simulink model "Trajektorienfolgeregelung_test"  (R2020a)
settings: Solver=ode1  StartTime=0.0  StopTime=3.5  FixedStep=0.01  RelTol=1e-10
undefined symbols (not defined in the file or in its folder): simparams
libraries: dspfdesign x3
settings Model: Creator=Frederik  LastModifiedBy=Frederik

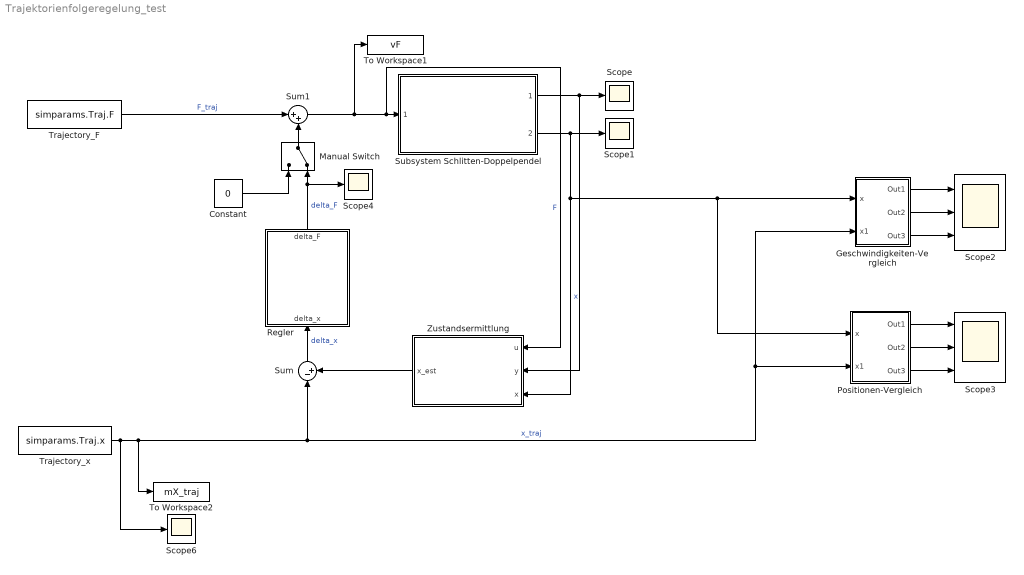
== system Trajektorienfolgeregelung_test ==
  Constant : Constant  Value=0
  Geschwindigkeiten-Vergleich : Subsystem
  Manual Switch : ManualSwitch  CurrentSetting=0
  Positionen-Vergleich : Subsystem
  Regler : Subsystem  mask{RegData=simparams.TrajRegDataF}
      mask prompts: RegData "TrajRegDataF"
  Scope{,1,4,6} (4 alike) : Scope
  Scope2 : Scope  NumInputPorts=3
  Scope3 : Scope  NumInputPorts=3
  Subsystem Schlitten-Doppelpendel : Subsystem  ReferencedSubsystem=SchlittenPendel  params=simparams.gesamtmodell.schlittenpendel
  Sum : Sum  Inputs=|-+
  Sum1 : Sum  Inputs=|++
  To Workspace1 : ToWorkspace  VariableName=vF  SaveFormat=Timeseries  SampleTime=-1
  To Workspace2 : ToWorkspace  VariableName=mX_traj  SaveFormat=Timeseries  SampleTime=-1
  Trajectory_F : FromWorkspace  VariableName=simparams.Traj.F  Interpolate=off  OutputAfterFinalValue=Setting to zero
  Trajectory_x : FromWorkspace  VariableName=simparams.Traj.x  Interpolate=off  OutputAfterFinalValue=Setting to zero
  Zustandsermittlung : Subsystem  Variant=on  VariantControl=Choice  PropagateVariantConditions=on  mask{BeoData=simparams.TrajRegDataF, xtype=Zustandsmessung}
      mask prompts: BeoData "Beobachter"; xtype "Zustandsermittlung"
      mask TypeOptions xtype: Zustandsmessung | Beobachter | Differenzieren
  wires:
  Subsystem Schlitten-Doppelpendel/1 -> Zustandsermittlung/2(y), Scope/1
  Trajectory_x/1 -> Sum/1, Positionen-Vergleich/2(x1), Geschwindigkeiten-Vergleich/2(x1), To Workspace2/1, Scope6/1  "x_traj"
  Trajectory_F/1 -> Sum1/1  "F_traj"
  Sum1/1 -> To Workspace1/1, Zustandsermittlung/1(u), Subsystem Schlitten-Doppelpendel/1  "F"
  Manual Switch/1 -> Sum1/2
  Constant/1 -> Manual Switch/1
  Sum/1 -> Regler/1(delta_x)  "delta_x"
  Regler/1(delta_F) -> Scope4/1, Manual Switch/2  "delta_F"
  Geschwindigkeiten-Vergleich/1(Out1) -> Scope2/1
  Geschwindigkeiten-Vergleich/2(Out2) -> Scope2/2
  Geschwindigkeiten-Vergleich/3(Out3) -> Scope2/3
  Positionen-Vergleich/1(Out1) -> Scope3/1
  Positionen-Vergleich/2(Out2) -> Scope3/2
  Positionen-Vergleich/3(Out3) -> Scope3/3
  Subsystem Schlitten-Doppelpendel/2 -> Zustandsermittlung/3(x), Positionen-Vergleich/1(x), Geschwindigkeiten-Vergleich/1(x), Scope1/1  "x"
  Zustandsermittlung/1(x_est) -> Sum/2

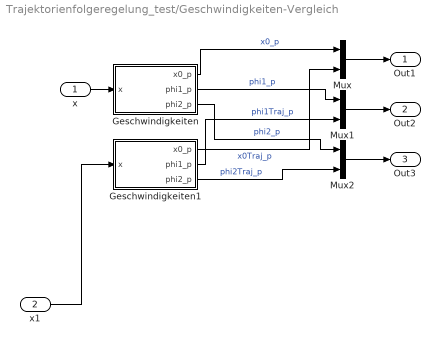
== system Trajektorienfolgeregelung_test/Geschwindigkeiten-Vergleich ==
  x : Inport
  x1 : Inport  Port=2
  Geschwindigkeiten : Subsystem
  Geschwindigkeiten1 : Subsystem
  Mux : Mux  Inputs=2
  Mux1 : Mux  Inputs=2
  Mux2 : Mux  Inputs=2
  Out1 : Outport
  Out2 : Outport  Port=2
  Out3 : Outport  Port=3
  wires:
  Geschwindigkeiten/1(x0_p) -> Mux/1  "x0_p"
  x/1 -> Geschwindigkeiten/1(x)
  Mux1/1 -> Out2/1
  Geschwindigkeiten1/2(phi1_p) -> Mux1/2  "phi1Traj_p"
  Geschwindigkeiten/3(phi2_p) -> Mux2/1  "phi2_p"
  Geschwindigkeiten1/3(phi2_p) -> Mux2/2  "phi2Traj_p"
  x1/1 -> Geschwindigkeiten1/1(x)
  Mux2/1 -> Out3/1
  Geschwindigkeiten1/1(x0_p) -> Mux/2  "x0Traj_p"
  Geschwindigkeiten/2(phi1_p) -> Mux1/1  "phi1_p"
  Mux/1 -> Out1/1

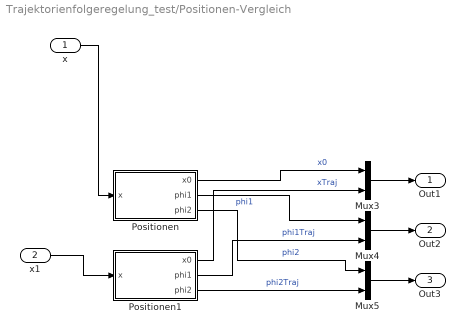
== system Trajektorienfolgeregelung_test/Positionen-Vergleich ==
  x : Inport
  x1 : Inport  Port=2
  Mux3 : Mux  Inputs=2
  Mux4 : Mux  Inputs=2
  Mux5 : Mux  Inputs=2
  Positionen : Subsystem
  Positionen1 : Subsystem
  Out1 : Outport
  Out2 : Outport  Port=2
  Out3 : Outport  Port=3
  wires:
  Positionen/3(phi2) -> Mux5/1  "phi2"
  Mux3/1 -> Out1/1
  Positionen1/3(phi2) -> Mux5/2  "phi2Traj"
  x1/1 -> Positionen1/1(x)
  Mux5/1 -> Out3/1
  Mux4/1 -> Out2/1
  Positionen1/1(x0) -> Mux3/2  "xTraj"
  Positionen1/2(phi1) -> Mux4/2  "phi1Traj"
  Positionen/1(x0) -> Mux3/1  "x0"
  Positionen/2(phi1) -> Mux4/1  "phi1"
  x/1 -> Positionen/1(x)

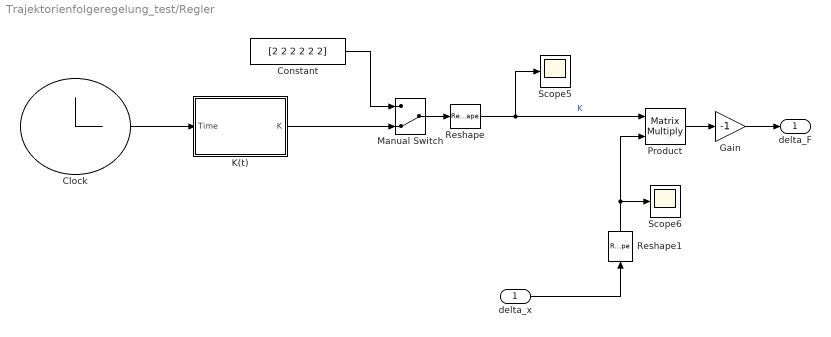
== system Trajektorienfolgeregelung_test/Regler ==
  delta_x : Inport
  Clock : Clock
  Constant : Constant  Value=[2 2 2 2 2 2]
  Gain : Gain  Gain=-1
  K(t) : Subsystem
  Manual Switch : ManualSwitch  CurrentSetting=0
  Product : Product  Multiplication=Matrix(*)
  Reshape : Reshape  OutputDimensionality=Row vector (2-D)
  Reshape1 : Reshape  OutputDimensionality=Column vector (2-D)
  Scope5 : Scope
  Scope6 : Scope
  delta_F : Outport
  wires:
  Product/1 -> Gain/1
  Reshape1/1 -> Product/2, Scope6/1
  Reshape/1 -> Scope5/1, Product/1  "K"
  delta_x/1 -> Reshape1/1
  Constant/1 -> Manual Switch/1
  Gain/1 -> delta_F/1
  Manual Switch/1 -> Reshape/1
  Clock/1 -> K(t)/1(Time)
  K(t)/1(K) -> Manual Switch/2

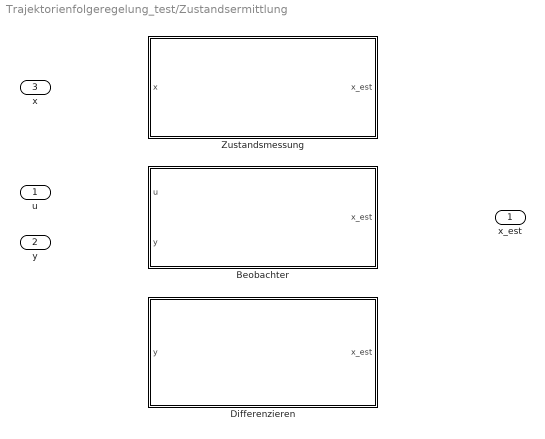
== system Trajektorienfolgeregelung_test/Zustandsermittlung ==
  u : Inport
  y : Inport  Port=2
  x : Inport  Port=3
  Beobachter : Subsystem  VariantControl=simparams.Zustandsermittlung==2
  Differenzieren : Subsystem  VariantControl=simparams.Zustandsermittlung==3
  Zustandsmessung : Subsystem  VariantControl=simparams.Zustandsermittlung==1
  x_est : Outport

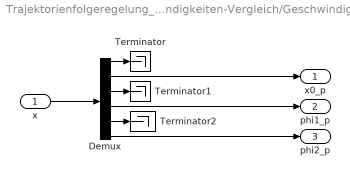
== system Trajektorienfolgeregelung_test/Geschwindigkeiten-Vergleich/Geschwindigkeiten ==
  x : Inport
  Demux : Demux  Outputs=6
  Terminator : Terminator
  Terminator1 : Terminator
  Terminator2 : Terminator
  x0_p : Outport
  phi1_p : Outport  Port=2
  phi2_p : Outport  Port=3
  wires:
  Demux/4 -> phi1_p/1
  Demux/2 -> x0_p/1
  Demux/5 -> Terminator2/1
  x/1 -> Demux/1
  Demux/3 -> Terminator1/1
  Demux/1 -> Terminator/1
  Demux/6 -> phi2_p/1

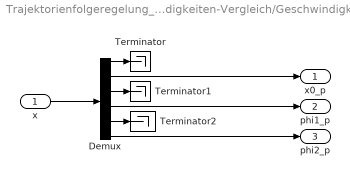
== system Trajektorienfolgeregelung_test/Geschwindigkeiten-Vergleich/Geschwindigkeiten1 ==
  x : Inport
  Demux : Demux  Outputs=6
  Terminator : Terminator
  Terminator1 : Terminator
  Terminator2 : Terminator
  x0_p : Outport
  phi1_p : Outport  Port=2
  phi2_p : Outport  Port=3
  wires:
  Demux/4 -> phi1_p/1
  Demux/2 -> x0_p/1
  Demux/5 -> Terminator2/1
  x/1 -> Demux/1
  Demux/3 -> Terminator1/1
  Demux/1 -> Terminator/1
  Demux/6 -> phi2_p/1

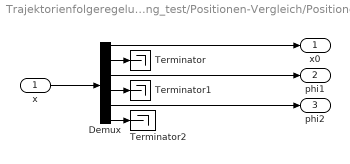
== system Trajektorienfolgeregelung_test/Positionen-Vergleich/Positionen ==
  x : Inport
  Demux : Demux  Outputs=6
  Terminator : Terminator
  Terminator1 : Terminator
  Terminator2 : Terminator
  x0 : Outport
  phi1 : Outport  Port=2
  phi2 : Outport  Port=3
  wires:
  Demux/3 -> phi1/1
  Demux/1 -> x0/1
  x/1 -> Demux/1
  Demux/5 -> phi2/1
  Demux/2 -> Terminator/1
  Demux/4 -> Terminator1/1
  Demux/6 -> Terminator2/1

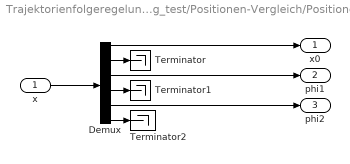
== system Trajektorienfolgeregelung_test/Positionen-Vergleich/Positionen1 ==
  x : Inport
  Demux : Demux  Outputs=6
  Terminator : Terminator
  Terminator1 : Terminator
  Terminator2 : Terminator
  x0 : Outport
  phi1 : Outport  Port=2
  phi2 : Outport  Port=3
  wires:
  Demux/3 -> phi1/1
  Demux/1 -> x0/1
  x/1 -> Demux/1
  Demux/5 -> phi2/1
  Demux/2 -> Terminator/1
  Demux/4 -> Terminator1/1
  Demux/6 -> Terminator2/1

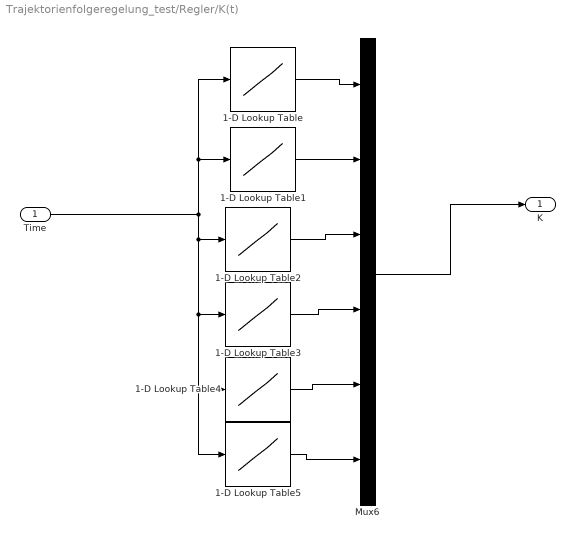
== system Trajektorienfolgeregelung_test/Regler/K(t) ==
  Time : Inport
  1-D Lookup Table : Lookup_n-D  NumberOfTableDimensions=1  BreakpointsForDimension1=RegData.T.data  Table=RegData.K.data(:,1)  InternalRulePriority=Speed  RndMeth=Simplest  InputSameDT=on
  1-D Lookup Table1 : Lookup_n-D  NumberOfTableDimensions=1  BreakpointsForDimension1=RegData.T.data  Table=RegData.K.data(:,2)  InternalRulePriority=Speed  RndMeth=Simplest  InputSameDT=on
  1-D Lookup Table2 : Lookup_n-D  NumberOfTableDimensions=1  BreakpointsForDimension1=RegData.T.data  Table=RegData.K.data(:,3)  InternalRulePriority=Speed  RndMeth=Simplest  InputSameDT=on
  1-D Lookup Table3 : Lookup_n-D  NumberOfTableDimensions=1  BreakpointsForDimension1=RegData.T.data  Table=RegData.K.data(:,4)  InternalRulePriority=Speed  RndMeth=Simplest  InputSameDT=on
  1-D Lookup Table4 : Lookup_n-D  NumberOfTableDimensions=1  BreakpointsForDimension1=RegData.T.data  Table=RegData.K.data(:,5)  InternalRulePriority=Speed  RndMeth=Simplest  InputSameDT=on
  1-D Lookup Table5 : Lookup_n-D  NumberOfTableDimensions=1  BreakpointsForDimension1=RegData.T.data  Table=RegData.K.data(:,6)  InternalRulePriority=Speed  RndMeth=Simplest  InputSameDT=on
  Mux6 : Mux  Inputs=6
  K : Outport
  wires:
  1-D Lookup Table5/1 -> Mux6/6
  1-D Lookup Table2/1 -> Mux6/3
  1-D Lookup Table/1 -> Mux6/1
  Time/1 -> 1-D Lookup Table/1, 1-D Lookup Table1/1, 1-D Lookup Table5/1, 1-D Lookup Table4/1, 1-D Lookup Table3/1, 1-D Lookup Table2/1
  1-D Lookup Table4/1 -> Mux6/5
  1-D Lookup Table3/1 -> Mux6/4
  Mux6/1 -> K/1
  1-D Lookup Table1/1 -> Mux6/2

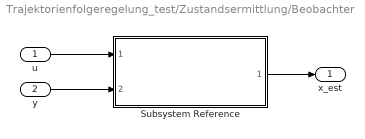
== system Trajektorienfolgeregelung_test/Zustandsermittlung/Beobachter ==
  u : Inport
  y : Inport  Port=2
  Subsystem Reference : Subsystem  ReferencedSubsystem=Beobachter  A=BeoData.A.data  B=BeoData.B.data  C=BeoData.C.data  L=BeoData.L.data  vT=[]  xb0=BeoData.xb0
  x_est : Outport
  wires:
  Subsystem Reference/1 -> x_est/1
  y/1 -> Subsystem Reference/2
  u/1 -> Subsystem Reference/1

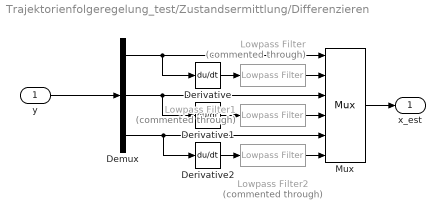
== system Trajektorienfolgeregelung_test/Zustandsermittlung/Differenzieren ==
  y : Inport
  Demux : Demux  Outputs=3
  Derivative : Derivative  CoefficientInTFapproximation=1
  Derivative1 : Derivative  CoefficientInTFapproximation=1
  Derivative2 : Derivative  CoefficientInTFapproximation=1
  Lowpass Filter : dspfdesign/Lowpass Filter  Commented=through  FilterType=FIR  DesignForMinimumOrder=on  FilterOrder=50  PassbandFrequency=25  StopbandFrequency=100  PassbandRipple=0.1  StopbandAttenuation=80  InheritSampleRate=off  SampleRate=1000  SimulateUsing=Interpreted execution  roundingMode=Floor  coeffsDataTypeStr=fixdt(1,16)
  Lowpass Filter1 : dspfdesign/Lowpass Filter  Commented=through  FilterType=FIR  DesignForMinimumOrder=on  FilterOrder=50  PassbandFrequency=25  StopbandFrequency=100  PassbandRipple=0.1  StopbandAttenuation=80  InheritSampleRate=off  SampleRate=1000  SimulateUsing=Interpreted execution  roundingMode=Floor  coeffsDataTypeStr=fixdt(1,16)
  Lowpass Filter2 : dspfdesign/Lowpass Filter  Commented=through  FilterType=FIR  DesignForMinimumOrder=on  FilterOrder=50  PassbandFrequency=25  StopbandFrequency=100  PassbandRipple=0.1  StopbandAttenuation=80  InheritSampleRate=off  SampleRate=1000  SimulateUsing=Interpreted execution  roundingMode=Floor  coeffsDataTypeStr=fixdt(1,16)
  Mux : Mux  Inputs=6
  x_est : Outport
  wires:
  Mux/1 -> x_est/1
  y/1 -> Demux/1
  Demux/1 -> Derivative/1, Mux/1
  Demux/2 -> Derivative1/1, Mux/3
  Demux/3 -> Derivative2/1, Mux/5
  Derivative/1 -> Lowpass Filter/1
  Derivative1/1 -> Lowpass Filter1/1
  Derivative2/1 -> Lowpass Filter2/1
  Lowpass Filter/1 -> Mux/2
  Lowpass Filter1/1 -> Mux/4
  Lowpass Filter2/1 -> Mux/6

== system Trajektorienfolgeregelung_test/Zustandsermittlung/Zustandsmessung ==
  x : Inport
  x_est : Outport
  wires:
  x/1 -> x_est/1
